simulink model "DDCU_wxt_v02_forA_LabviewV03"  (R2014a)
settings: Solver=FixedStepDiscrete  StartTime=0.0  StopTime=50  FixedStep=0.0005  RelTol=1e-3
InitFcn:
  | Veh_Par_wxt
values from neighbouring files (symbols this model uses):
  ag_thr = 0.4*g    (= 3.924)    [Veh_Par_wxt.m]
  B = 2.25    [Veh_Par_wxt.m]
  bra_pre_em = 12    [Veh_Par_wxt.m]
  bra_pre_gz2 = 12/3    (= 4)    [Veh_Par_wxt.m]
  bra_pre_gz34 = 12/3    (= 4)    [Veh_Par_wxt.m]
  bra_pre_yd = 12/2    (= 6)    [Veh_Par_wxt.m]
  brakepre_dem_data = [0 1 2 3 4 5 6 7 8 9 10 11 12]    [Veh_Par_wxt.m]
  brakeTrq_dem_data = [0 218.198 436.396 654.594 872.792 1090.99 1309.188 1527.386 1745.584 1963.782 2181.98 2400.178 2618.376]    [Veh_Par_wxt.m]
  bratrq_max = 4*2618.376    (= 10473.504)    [Veh_Par_wxt.m]
  eff_tran = 0.75    [Veh_Par_wxt.m]
  G = Mass*g    (= 36297)    [Veh_Par_wxt.m]
  kd1 = 1    [Veh_Par_wxt.m]
  kd2 = 1    [Veh_Par_wxt.m]
  kd3 = 1    [Veh_Par_wxt.m]
  ki1 = 1    [Veh_Par_wxt.m]
  ki2 = 1    [Veh_Par_wxt.m]
  ki3 = 1    [Veh_Par_wxt.m]
  kp1 = 1    [Veh_Par_wxt.m]
  kp2 = 1    [Veh_Par_wxt.m]
  kp3 = 1    [Veh_Par_wxt.m]
  L = 3.12    [Veh_Par_wxt.m]
  premax = 12    [Veh_Par_wxt.m]
  Radius = 0.20    (= 0.2)    [Veh_Par_wxt.m]
  s_opt_yi_add = 0.05    [Veh_Par_wxt.m]
  s_opt_zhuan_add = 0.05    [Veh_Par_wxt.m]
  spd_map_mot = [0 100 200 300 360 400 500 600 700 800 900]*tras_ratio    [Veh_Par_wxt.m]
  spdmax = 900*tras_ratio    (= 5580)    [Veh_Par_wxt.m]
  speed_thr_park = 5/3.6/Radius*30/pi    (= 66.3145596216)    [Veh_Par_wxt.m]
  tras_ratio = 6.2    [Veh_Par_wxt.m]
  trq_map_mot = [1200 1200 1200 1200 1200 1080 864 720 617 540 480]/tras_ratio    [Veh_Par_wxt.m]
  trqmax = 80    [Veh_Par_wxt.m]
  trqmax_yd = 200    [Veh_Par_wxt.m]
  v_thr1_b = 5    [Veh_Par_wxt.m]
  v_thr2_b = 20    [Veh_Par_wxt.m]
  v_thr_park = 5    [Veh_Par_wxt.m]
undefined symbols (not defined in the file or in its folder): DiscIntNeverNeededParam
libraries: simulink x231, ec5744lib x19
(part 11 of 16)

== system DDCU_wxt_v02_forA_LabviewV03/Data_Input/MCU2_VCU1/MCU2_VCU1/M3InputVolt_Sub ==
  In1 : Inport
  Out1 : Outport
  wires:
  In1/1 -> Out1/1

== system DDCU_wxt_v02_forA_LabviewV03/Data_Input/MCU2_VCU1/MCU2_VCU1/M3Speed_Sub ==
  In1 : Inport
  Out1 : Outport
  wires:
  In1/1 -> Out1/1

== system DDCU_wxt_v02_forA_LabviewV03/Data_Input/MCU2_VCU1/MCU2_VCU1/M3State_Sub ==
  In1 : Inport
  Out1 : Outport
  wires:
  In1/1 -> Out1/1

== system DDCU_wxt_v02_forA_LabviewV03/Data_Input/MCU2_VCU1/MCU2_VCU1/M3Torque_Sub ==
  In1 : Inport
  Out1 : Outport
  wires:
  In1/1 -> Out1/1

== system DDCU_wxt_v02_forA_LabviewV03/Data_Input/MCU2_VCU2/MCU2_VCU2/M3FaultCode_Sub ==
  In1 : Inport
  Out1 : Outport
  wires:
  In1/1 -> Out1/1

== system DDCU_wxt_v02_forA_LabviewV03/Data_Input/MCU2_VCU2/MCU2_VCU2/M3FaultGrade_Sub ==
  In1 : Inport
  Out1 : Outport
  wires:
  In1/1 -> Out1/1

== system DDCU_wxt_v02_forA_LabviewV03/Data_Input/MCU2_VCU2/MCU2_VCU2/M3IGBTTemp_Sub ==
  In1 : Inport
  Out1 : Outport
  wires:
  In1/1 -> Out1/1

== system DDCU_wxt_v02_forA_LabviewV03/Data_Input/MCU2_VCU2/MCU2_VCU2/M3Temp_Sub ==
  In1 : Inport
  Out1 : Outport
  wires:
  In1/1 -> Out1/1

== system DDCU_wxt_v02_forA_LabviewV03/Data_Input/MCU2_VCU2/MCU2_VCU2/M3TqLimit_Sub ==
  In1 : Inport
  Out1 : Outport
  wires:
  In1/1 -> Out1/1

== system DDCU_wxt_v02_forA_LabviewV03/Data_Input/MCU2_VCU3/MCU2_VCU3/M4Current_Sub ==
  In1 : Inport
  Out1 : Outport
  wires:
  In1/1 -> Out1/1

== system DDCU_wxt_v02_forA_LabviewV03/Data_Input/MCU2_VCU3/MCU2_VCU3/M4Direction_Sub ==
  In1 : Inport
  Out1 : Outport
  wires:
  In1/1 -> Out1/1

== system DDCU_wxt_v02_forA_LabviewV03/Data_Input/MCU2_VCU3/MCU2_VCU3/M4HeartBeat_Sub ==
  In1 : Inport
  Out1 : Outport
  wires:
  In1/1 -> Out1/1

== system DDCU_wxt_v02_forA_LabviewV03/Data_Input/MCU2_VCU3/MCU2_VCU3/M4InputVolt_Sub ==
  In1 : Inport
  Out1 : Outport
  wires:
  In1/1 -> Out1/1

== system DDCU_wxt_v02_forA_LabviewV03/Data_Input/MCU2_VCU3/MCU2_VCU3/M4Speed_Sub ==
  In1 : Inport
  Out1 : Outport
  wires:
  In1/1 -> Out1/1

== system DDCU_wxt_v02_forA_LabviewV03/Data_Input/MCU2_VCU3/MCU2_VCU3/M4State_Sub ==
  In1 : Inport
  Out1 : Outport
  wires:
  In1/1 -> Out1/1

== system DDCU_wxt_v02_forA_LabviewV03/Data_Input/MCU2_VCU3/MCU2_VCU3/M4Torque_Sub ==
  In1 : Inport
  Out1 : Outport
  wires:
  In1/1 -> Out1/1

== system DDCU_wxt_v02_forA_LabviewV03/Data_Input/MCU2_VCU4/MCU2_VCU4/M4FaultCode_Sub ==
  In1 : Inport
  Out1 : Outport
  wires:
  In1/1 -> Out1/1

== system DDCU_wxt_v02_forA_LabviewV03/Data_Input/MCU2_VCU4/MCU2_VCU4/M4FaultGrade_Sub ==
  In1 : Inport
  Out1 : Outport
  wires:
  In1/1 -> Out1/1

== system DDCU_wxt_v02_forA_LabviewV03/Data_Input/MCU2_VCU4/MCU2_VCU4/M4IGBTTemp_Sub ==
  In1 : Inport
  Out1 : Outport
  wires:
  In1/1 -> Out1/1

== system DDCU_wxt_v02_forA_LabviewV03/Data_Input/MCU2_VCU4/MCU2_VCU4/M4Temp_Sub ==
  In1 : Inport
  Out1 : Outport
  wires:
  In1/1 -> Out1/1

== system DDCU_wxt_v02_forA_LabviewV03/Data_Input/MCU2_VCU4/MCU2_VCU4/M4TqLimit_Sub ==
  In1 : Inport
  Out1 : Outport
  wires:
  In1/1 -> Out1/1

== system DDCU_wxt_v02_forA_LabviewV03/MainControl/mode_control/Park/park ==
  Signals : Inport
  1-D Lookup Table : Lookup_n-D  NumberOfTableDimensions=1  BreakpointsForDimension1=brakeTrq_dem_data  Table=brakepre_dem_data  InternalRulePriority=Speed  RndMeth=Simplest  InputSameDT=on
  1-D Lookup Table1 : Lookup_n-D  NumberOfTableDimensions=1  BreakpointsForDimension1=brakeTrq_dem_data  Table=brakepre_dem_data  InternalRulePriority=Speed  RndMeth=Simplest  InputSameDT=on
  Bus Selector : BusSelector  OutputSignals=YaoKong.brake_dem
  Constant : Constant  Value=bratrq_max
  Gain : Gain  Gain=1/2
  Gain1 : Gain  Gain=1/100
  Gain2 : Gain  Gain=1/2
  Gain3 : Gain  Gain=1/2
  HeartBeat : MATLAB Function  TreatAsAtomicUnit=on
  HeartBeat1 : MATLAB Function  TreatAsAtomicUnit=on
  Memory : Memory  InheritSampleTime=on
  Memory1 : Memory  InheritSampleTime=on
  Mux : Mux  Inputs=8
  Mux1 : Mux  Inputs=8
  Mux2 : Mux  Inputs=7
  Mux3 : Mux  Inputs=7
  Product : Product
  Saturation1 : Saturate  UpperLimit=premax  LowerLimit=0
  Saturation4 : Saturate  UpperLimit=premax  LowerLimit=0
  SpdLim_dem{,1..3} (4 alike) : Constant  Value=spdmax
  SpdSet_dem : Constant  Value=0
  SpdSet_dem1 : Constant
  SpdSet_dem2 : Constant
  SpdSet_dem3 : Constant
  TrqLim_dem{,1..3} (4 alike) : Constant
  TrqSet_dem{,1..3} (4 alike) : Constant  Value=0
  mot_drive : Constant
  mot_drive1 : Constant  Value=2
  mot_drive2 : Constant
  mot_drive3 : Constant  Value=2
  mot_enable{,1..3} (4 alike) : Constant  Value=2
  mot_mode{,1..3} (4 alike) : Constant
  mot_lf : Outport
  mot_lr : Outport  Port=2
  mot_rf : Outport  Port=3
  mot_rr : Outport  Port=4
  bra_pre_l : Outport  Port=5
  bra_pre_r : Outport  Port=6
  wires:
  mot_drive/1 -> Mux/3
  mot_mode/1 -> Mux/2
  TrqSet_dem/1 -> Mux/4
  mot_enable/1 -> Mux/1
  SpdSet_dem/1 -> Mux/5
  Mux/1 -> mot_lf/1
  Signals/1 -> Bus Selector/1
  1-D Lookup Table/1 -> Saturation4/1
  TrqLim_dem/1 -> Mux/6
  HeartBeat/1(life) -> Mux/8, Memory/1
  Memory/1 -> HeartBeat/1(life_pre)
  SpdLim_dem/1 -> Mux/7
  mot_drive1/1 -> Mux2/3
  mot_mode2/1 -> Mux2/2
  TrqSet_dem1/1 -> Mux2/4
  mot_enable2/1 -> Mux2/1
  SpdSet_dem1/1 -> Mux2/5
  Mux2/1 -> mot_rf/1
  TrqLim_dem1/1 -> Mux2/6
  SpdLim_dem1/1 -> Mux2/7
  mot_drive2/1 -> Mux1/3
  mot_mode1/1 -> Mux1/2
  TrqSet_dem2/1 -> Mux1/4
  mot_enable1/1 -> Mux1/1
  SpdSet_dem2/1 -> Mux1/5
  Mux1/1 -> mot_lr/1
  TrqLim_dem2/1 -> Mux1/6
  HeartBeat1/1(life) -> Mux1/8, Memory1/1
  Memory1/1 -> HeartBeat1/1(life_pre)
  SpdLim_dem2/1 -> Mux1/7
  mot_drive3/1 -> Mux3/3
  mot_mode3/1 -> Mux3/2
  TrqSet_dem3/1 -> Mux3/4
  mot_enable3/1 -> Mux3/1
  SpdSet_dem3/1 -> Mux3/5
  Mux3/1 -> mot_rr/1
  TrqLim_dem3/1 -> Mux3/6
  SpdLim_dem3/1 -> Mux3/7
  Constant/1 -> Product/1
  Bus Selector/1 -> Gain1/1  "<brake_dem>"
  Product/1 -> Gain/1
  Gain/1 -> Gain3/1, Gain2/1
  Gain1/1 -> Product/2
  Gain2/1 -> 1-D Lookup Table/1
  Gain3/1 -> 1-D Lookup Table1/1
  1-D Lookup Table1/1 -> Saturation1/1
  Saturation4/1 -> bra_pre_l/1
  Saturation1/1 -> bra_pre_r/1

== system DDCU_wxt_v02_forA_LabviewV03/MainControl/mode_control/backward/backward ==
  Signals : Inport
  Brake : Subsystem  TreatAsAtomicUnit=on
  Bus Selector : BusSelector  OutputSignals=YaoKong.acc_dem,YaoKong.brake_dem,YaoKong.HAC
  Constant : Constant  Value=0.15
  Drive : Subsystem  TreatAsAtomicUnit=on
  MATLAB Function : MATLAB Function  TreatAsAtomicUnit=on
  Multiport Switch : MultiPortSwitch  DataPortOrder=Zero-based contiguous  Inputs=2
  Switch Case1 : SwitchCase  CaseConditions={0,1}  ShowDefaultCase=off
  backward_dem : Outport
  wires:
  Constant/1 -> Brake/2(s_opt_yi)
  Brake/1(backward_dem) -> Multiport Switch/3
  Drive/1(backward_dem) -> Multiport Switch/2
  MATLAB Function/1(y) -> Switch Case1/1, Multiport Switch/1
  Switch Case1/2 -> Brake/Action
  Switch Case1/1 -> Drive/Action
  Multiport Switch/1 -> backward_dem/1
  Signals/1 -> Bus Selector/1, Drive/1(Signals), Brake/1(Signals)
  Bus Selector/1 -> MATLAB Function/1(acc_dem)  "<acc_dem>"
  Bus Selector/2 -> MATLAB Function/2(brake_dem)  "<brake_dem>"
  Bus Selector/3 -> MATLAB Function/3(HAC)  "<HAC>"

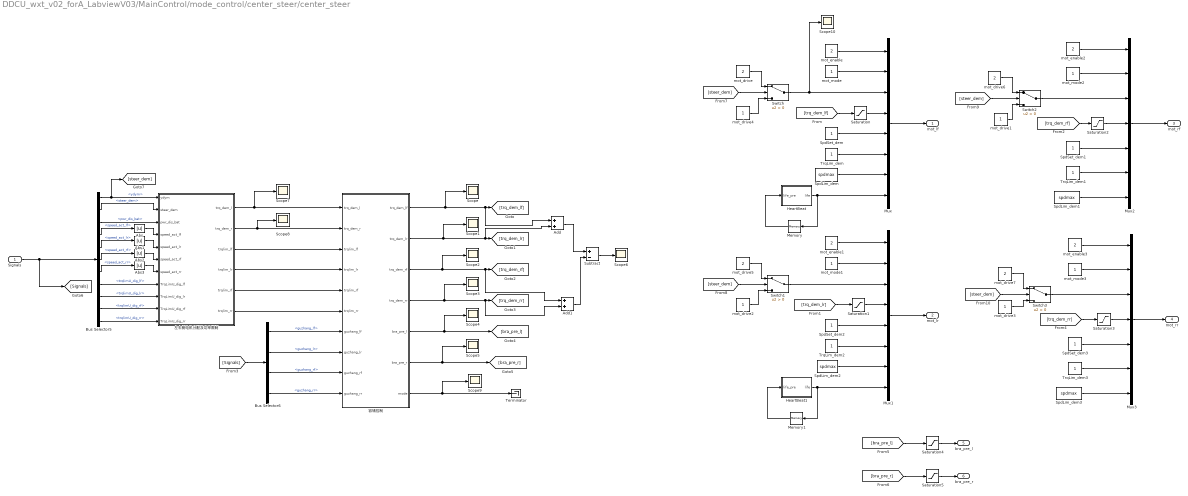
== system DDCU_wxt_v02_forA_LabviewV03/MainControl/mode_control/center_steer/center_steer ==
  Signals : Inport
  Abs{,1..3} (4 alike) : Abs
  Add : Sum
  Add1 : Sum
  Bus Selector5 : BusSelector  OutputSignals=ydym,YaoKong.steer_dem,Bat.pwr_dis_bat,DriveMotor.speed_act_lf,DriveMotor.speed_act_lr,DriveMotor.speed_act_rf,DriveMotor.speed_act_rr,DriveMotor.trqlimU_dig_lf,DriveMotor.trqlimU_dig_lr,DriveMotor.trqlimU_dig_rf,DriveMotor.trqlimU_dig_rr
  Bus Selector6 : BusSelector  OutputSignals=DriveMotor.guzhang_lf,DriveMotor.guzhang_lr,DriveMotor.guzhang_rf,DriveMotor.guzhang_rr
  HeartBeat : MATLAB Function  TreatAsAtomicUnit=on
  HeartBeat1 : MATLAB Function  TreatAsAtomicUnit=on
  Memory : Memory  InheritSampleTime=on
  Memory1 : Memory  InheritSampleTime=on
  Mux : Mux  Inputs=8
  Mux1 : Mux  Inputs=8
  Mux2 : Mux  Inputs=7
  Mux3 : Mux  Inputs=7
  Saturation{,1..3} (4 alike) : Saturate  UpperLimit=trqmax_yd  LowerLimit=0
  Saturation4 : Saturate  UpperLimit=premax  LowerLimit=0
  Saturation5 : Saturate  UpperLimit=premax  LowerLimit=0
  Scope{,1..10} (11 alike) : Scope
      Scope settings: SaveName=ScopeData47
      Scope1 settings: SaveName=ScopeData48
      Scope10 settings: SaveName=ScopeData58
      Scope2 settings: SaveName=ScopeData49
      Scope3 settings: SaveName=ScopeData50
      Scope4 settings: SaveName=ScopeData51
      Scope5 settings: SaveName=ScopeData52
      Scope6 settings: SaveName=ScopeData54
      Scope7 settings: SaveName=ScopeData55
      Scope8 settings: SaveName=ScopeData56
      Scope9 settings: SaveName=ScopeData57
  SpdLim_dem{,1..3} (4 alike) : Constant  Value=spdmax
  SpdSet_dem{,1..3} (4 alike) : Constant
  Subtract : Sum  Inputs=+-
  Switch{,1..3} (4 alike) : Switch  Criteria=u2 > Threshold
  Terminator : Terminator
  TrqLim_dem{,1..3} (4 alike) : Constant
  mot_drive{,5..7} (4 alike) : Constant  Value=2
  mot_drive{1..4} (4 alike) : Constant
  mot_enable{,1..3} (4 alike) : Constant  Value=2
  mot_mode{,1..3} (4 alike) : Constant
  容错控制 : Subsystem
  左右侧电机分配及功率限制 : Subsystem
  mot_lf : Outport
  mot_lr : Outport  Port=2
  mot_rf : Outport  Port=3
  mot_rr : Outport  Port=4
  bra_pre_l : Outport  Port=5
  bra_pre_r : Outport  Port=6
  wires:
  Signals/1 -> [Signals], Bus Selector5/1
  Bus Selector5/3 -> 左右侧电机分配及功率限制/3(pwr_dis_bat)  "<pwr_dis_bat>"
  Bus Selector5/4 -> Abs/1  "<speed_act_lf>"
  Bus Selector5/5 -> Abs1/1  "<speed_act_lr>"
  Bus Selector5/6 -> Abs2/1  "<speed_act_rf>"
  Bus Selector5/7 -> Abs3/1  "<speed_act_rr>"
  Bus Selector5/11 -> 左右侧电机分配及功率限制/11(TrqLimU_dig_rr)  "<trqlimU_dig_rr>"
  Bus Selector5/10 -> 左右侧电机分配及功率限制/10(TrqLimU_dig_rf)  "<trqlimU_dig_rf>"
  Bus Selector5/8 -> 左右侧电机分配及功率限制/8(TrqLimU_dig_lf)  "<trqlimU_dig_lf>"
  Bus Selector5/9 -> 左右侧电机分配及功率限制/9(TrqLimU_dig_lr)  "<trqlimU_dig_lr>"
  [Signals] -> Bus Selector6/1
  左右侧电机分配及功率限制/2(trq_dem_r) -> Scope8/1, 容错控制/2(trq_dem_r)
  左右侧电机分配及功率限制/1(trq_dem_l) -> Scope7/1, 容错控制/1(trq_dem_l)
  Bus Selector6/4 -> 容错控制/10(guzhang_rr)  "<guzhang_rr>"
  Bus Selector6/3 -> 容错控制/9(guzhang_rf)  "<guzhang_rf>"
  Bus Selector6/2 -> 容错控制/8(guzhang_lr)  "<guzhang_lr>"
  Bus Selector6/1 -> 容错控制/7(guzhang_lf)  "<guzhang_lf>"
  左右侧电机分配及功率限制/5(trqlim_rf) -> 容错控制/5(trqlim_rf)
  左右侧电机分配及功率限制/4(trqlim_lr) -> 容错控制/4(trqlim_lr)
  左右侧电机分配及功率限制/6(trqlim_rr) -> 容错控制/6(trqlim_rr)
  左右侧电机分配及功率限制/3(trqlim_lf) -> 容错控制/3(trqlim_lf)
  Bus Selector5/2 -> 左右侧电机分配及功率限制/2(steer_dem)  "<steer_dem>"
  容错控制/1(trq_dem_lf) -> Scope/1, Add/1, [trq_dem_lf]
  容错控制/3(trq_dem_rf) -> Scope2/1, Add1/1, [trq_dem_rf]
  容错控制/4(trq_dem_rr) -> Scope3/1, Add1/2, [trq_dem_rr]
  容错控制/5(bra_pre_l) -> Scope4/1, [bra_pre_l]
  容错控制/6(bra_pre_r) -> Scope5/1, [bra_pre_r]
  容错控制/2(trq_dem_lr) -> Scope1/1, Add/2, [trq_dem_lr]
  Switch/1 -> Scope10/1, Mux/3
  mot_mode/1 -> Mux/2
  [trq_dem_lf] -> Saturation/1
  mot_enable/1 -> Mux/1
  SpdSet_dem/1 -> Mux/5
  Mux/1 -> mot_lf/1
  TrqLim_dem/1 -> Mux/6
  HeartBeat/1(life) -> Mux/8, Memory/1
  Memory/1 -> HeartBeat/1(life_pre)
  SpdLim_dem/1 -> Mux/7
  Switch2/1 -> Mux2/3
  mot_mode2/1 -> Mux2/2
  [trq_dem_rf] -> Saturation2/1
  mot_enable2/1 -> Mux2/1
  SpdSet_dem1/1 -> Mux2/5
  Mux2/1 -> mot_rf/1
  TrqLim_dem1/1 -> Mux2/6
  SpdLim_dem1/1 -> Mux2/7
  Switch1/1 -> Mux1/3
  mot_mode1/1 -> Mux1/2
  [trq_dem_lr] -> Saturation1/1
  mot_enable1/1 -> Mux1/1
  SpdSet_dem2/1 -> Mux1/5
  Mux1/1 -> mot_lr/1
  TrqLim_dem2/1 -> Mux1/6
  HeartBeat1/1(life) -> Mux1/8, Memory1/1
  Memory1/1 -> HeartBeat1/1(life_pre)
  SpdLim_dem2/1 -> Mux1/7
  Switch3/1 -> Mux3/3
  mot_mode3/1 -> Mux3/2
  [trq_dem_rr] -> Saturation3/1
  mot_enable3/1 -> Mux3/1
  SpdSet_dem3/1 -> Mux3/5
  Mux3/1 -> mot_rr/1
  TrqLim_dem3/1 -> Mux3/6
  SpdLim_dem3/1 -> Mux3/7
  [bra_pre_l] -> Saturation4/1
  [bra_pre_r] -> Saturation5/1
  Saturation/1 -> Mux/4
  Saturation1/1 -> Mux1/4
  Saturation2/1 -> Mux2/4
  Saturation3/1 -> Mux3/4
  Saturation4/1 -> bra_pre_l/1
  Saturation5/1 -> bra_pre_r/1
  Add/1 -> Subtract/1
  Add1/1 -> Subtract/2
  Subtract/1 -> Scope6/1
  容错控制/7(mode) -> Terminator/1, Scope9/1
  Abs/1 -> 左右侧电机分配及功率限制/4(speed_act_lf)
  Abs1/1 -> 左右侧电机分配及功率限制/5(speed_act_lr)
  Abs2/1 -> 左右侧电机分配及功率限制/6(speed_act_rf)
  Abs3/1 -> 左右侧电机分配及功率限制/7(speed_act_rr)
  [steer_dem] -> Switch/2
  mot_drive4/1 -> Switch/3
  mot_drive/1 -> Switch/1
  [steer_dem] -> Switch1/2
  mot_drive5/1 -> Switch1/1
  mot_drive2/1 -> Switch1/3
  [steer_dem] -> Switch2/2
  mot_drive6/1 -> Switch2/1
  mot_drive1/1 -> Switch2/3
  [steer_dem] -> Switch3/2
  mot_drive7/1 -> Switch3/1
  mot_drive3/1 -> Switch3/3
  Bus Selector5/1 -> [steer_dem], 左右侧电机分配及功率限制/1(ydym)  "<ydym>"

== system DDCU_wxt_v02_forA_LabviewV03/MainControl/mode_control/emergency_stop/emergency_stop ==
  Signals : Inport
  Bus Selector : BusSelector  OutputSignals=YaoKong.brake_dem
  Constant : Constant  Value=bra_pre_em
  HeartBeat : MATLAB Function  TreatAsAtomicUnit=on
  HeartBeat1 : MATLAB Function  TreatAsAtomicUnit=on
  Memory : Memory  InheritSampleTime=on
  Memory1 : Memory  InheritSampleTime=on
  Mux : Mux  Inputs=8
  Mux1 : Mux  Inputs=8
  Mux2 : Mux  Inputs=7
  Mux3 : Mux  Inputs=7
  Saturation1 : Saturate  UpperLimit=premax  LowerLimit=0
  Saturation4 : Saturate  UpperLimit=premax  LowerLimit=0
  SpdLim_dem{,1..3} (4 alike) : Constant  Value=spdmax
  SpdSet_dem{,1..3} (4 alike) : Constant
  Terminator : Terminator
  TrqLim_dem{,1..3} (4 alike) : Constant
  TrqSet_dem{,1..3} (4 alike) : Constant  Value=0
  mot_drive : Constant
  mot_drive1 : Constant  Value=2
  mot_drive2 : Constant
  mot_drive3 : Constant  Value=2
  mot_enable{,1..3} (4 alike) : Constant  Value=2
  mot_mode{,1..3} (4 alike) : Constant
  mot_lf : Outport
  mot_lr : Outport  Port=2
  mot_rf : Outport  Port=3
  mot_rr : Outport  Port=4
  bra_pre_l : Outport  Port=5
  bra_pre_r : Outport  Port=6
  wires:
  mot_drive/1 -> Mux/3
  mot_mode/1 -> Mux/2
  TrqSet_dem/1 -> Mux/4
  mot_enable/1 -> Mux/1
  SpdSet_dem/1 -> Mux/5
  Mux/1 -> mot_lf/1
  Signals/1 -> Bus Selector/1
  Bus Selector/1 -> Terminator/1  "<brake_dem>"
  TrqLim_dem/1 -> Mux/6
  HeartBeat/1(life) -> Mux/8, Memory/1
  Memory/1 -> HeartBeat/1(life_pre)
  SpdLim_dem/1 -> Mux/7
  mot_drive1/1 -> Mux2/3
  mot_mode2/1 -> Mux2/2
  TrqSet_dem1/1 -> Mux2/4
  mot_enable2/1 -> Mux2/1
  SpdSet_dem1/1 -> Mux2/5
  Mux2/1 -> mot_rf/1
  TrqLim_dem1/1 -> Mux2/6
  SpdLim_dem1/1 -> Mux2/7
  mot_drive2/1 -> Mux1/3
  mot_mode1/1 -> Mux1/2
  TrqSet_dem2/1 -> Mux1/4
  mot_enable1/1 -> Mux1/1
  SpdSet_dem2/1 -> Mux1/5
  Mux1/1 -> mot_lr/1
  TrqLim_dem2/1 -> Mux1/6
  HeartBeat1/1(life) -> Mux1/8, Memory1/1
  Memory1/1 -> HeartBeat1/1(life_pre)
  SpdLim_dem2/1 -> Mux1/7
  mot_drive3/1 -> Mux3/3
  mot_mode3/1 -> Mux3/2
  TrqSet_dem3/1 -> Mux3/4
  mot_enable3/1 -> Mux3/1
  SpdSet_dem3/1 -> Mux3/5
  Mux3/1 -> mot_rr/1
  TrqLim_dem3/1 -> Mux3/6
  SpdLim_dem3/1 -> Mux3/7
  Constant/1 -> Saturation4/1, Saturation1/1
  Saturation4/1 -> bra_pre_l/1
  Saturation1/1 -> bra_pre_r/1

== system DDCU_wxt_v02_forA_LabviewV03/MainControl/mode_control/forward/forward ==
  note: 最佳滑移率
  note: 再加一些滤波的措施
  note: 坡道驻车，目前一直给1
  Signals : Inport
  Brake : Subsystem  TreatAsAtomicUnit=on
  Bus Selector : BusSelector  OutputSignals=YaoKong.acc_dem,YaoKong.brake_dem,YaoKong.HAC
  Constant : Constant  Value=0.15  SampleTime=-1
  Drive : Subsystem  TreatAsAtomicUnit=on
  MATLAB Function : MATLAB Function  TreatAsAtomicUnit=on
  Multiport Switch : MultiPortSwitch  DataPortOrder=Zero-based contiguous  Inputs=2
  Switch Case1 : SwitchCase  CaseConditions={0,1}  ShowDefaultCase=off
  forward_dem : Outport
  wires:
  Signals/1 -> Brake/1(Signals), Drive/1(Signals), Bus Selector/1
  Multiport Switch/1 -> forward_dem/1
  Switch Case1/1 -> Drive/Action
  Switch Case1/2 -> Brake/Action
  Bus Selector/1 -> MATLAB Function/1(acc_dem)  "<acc_dem>"
  MATLAB Function/1(y) -> Multiport Switch/1, Switch Case1/1
  Drive/1(forward_dem) -> Multiport Switch/2
  Brake/1(forward_dem) -> Multiport Switch/3
  Constant/1 -> Brake/2(s_opt_yi)
  Bus Selector/2 -> MATLAB Function/2(brake_dem)  "<brake_dem>"
  Bus Selector/3 -> MATLAB Function/3(HAC)  "<HAC>"

== system DDCU_wxt_v02_forA_LabviewV03/MainControl/mode_control/neutral/neutral ==
  Signals : Inport
  Bus Selector : BusSelector  OutputSignals=YaoKong.brake_dem
  Constant : Constant  Value=0
  Gain : Gain  Gain=1/2
  HeartBeat : MATLAB Function  TreatAsAtomicUnit=on
  HeartBeat1 : MATLAB Function  TreatAsAtomicUnit=on
  Memory : Memory  InheritSampleTime=on
  Memory1 : Memory  InheritSampleTime=on
  Mux : Mux  Inputs=8
  Mux1 : Mux  Inputs=8
  Mux2 : Mux  Inputs=7
  Mux3 : Mux  Inputs=7
  SpdLim_dem{,1..3} (4 alike) : Constant  Value=spdmax
  SpdSet_dem{,1..3} (4 alike) : Constant
  Terminator : Terminator
  TrqLim_dem{,1..3} (4 alike) : Constant
  TrqSet_dem{,1..3} (4 alike) : Constant  Value=0
  mot_drive : Constant
  mot_drive1 : Constant  Value=2
  mot_drive2 : Constant
  mot_drive3 : Constant  Value=2
  mot_enable{,1..3} (4 alike) : Constant  Value=2
  mot_mode{,1..3} (4 alike) : Constant
  mot_lf : Outport
  mot_lr : Outport  Port=2
  mot_rf : Outport  Port=3
  mot_rr : Outport  Port=4
  bra_pre_l : Outport  Port=5
  bra_pre_r : Outport  Port=6
  wires:
  mot_drive/1 -> Mux/3
  mot_mode/1 -> Mux/2
  TrqSet_dem/1 -> Mux/4
  mot_enable/1 -> Mux/1
  SpdSet_dem/1 -> Mux/5
  Mux/1 -> mot_lf/1
  Signals/1 -> Bus Selector/1
  Bus Selector/1 -> Gain/1  "<brake_dem>"
  TrqLim_dem/1 -> Mux/6
  HeartBeat/1(life) -> Mux/8, Memory/1
  Memory/1 -> HeartBeat/1(life_pre)
  SpdLim_dem/1 -> Mux/7
  mot_drive1/1 -> Mux2/3
  mot_mode2/1 -> Mux2/2
  TrqSet_dem1/1 -> Mux2/4
  mot_enable2/1 -> Mux2/1
  SpdSet_dem1/1 -> Mux2/5
  Mux2/1 -> mot_rf/1
  TrqLim_dem1/1 -> Mux2/6
  SpdLim_dem1/1 -> Mux2/7
  mot_drive2/1 -> Mux1/3
  mot_mode1/1 -> Mux1/2
  TrqSet_dem2/1 -> Mux1/4
  mot_enable1/1 -> Mux1/1
  SpdSet_dem2/1 -> Mux1/5
  Mux1/1 -> mot_lr/1
  TrqLim_dem2/1 -> Mux1/6
  HeartBeat1/1(life) -> Mux1/8, Memory1/1
  Memory1/1 -> HeartBeat1/1(life_pre)
  SpdLim_dem2/1 -> Mux1/7
  mot_drive3/1 -> Mux3/3
  mot_mode3/1 -> Mux3/2
  TrqSet_dem3/1 -> Mux3/4
  mot_enable3/1 -> Mux3/1
  SpdSet_dem3/1 -> Mux3/5
  Mux3/1 -> mot_rr/1
  TrqLim_dem3/1 -> Mux3/6
  SpdLim_dem3/1 -> Mux3/7
  Gain/1 -> Terminator/1
  Constant/1 -> bra_pre_r/1, bra_pre_l/1

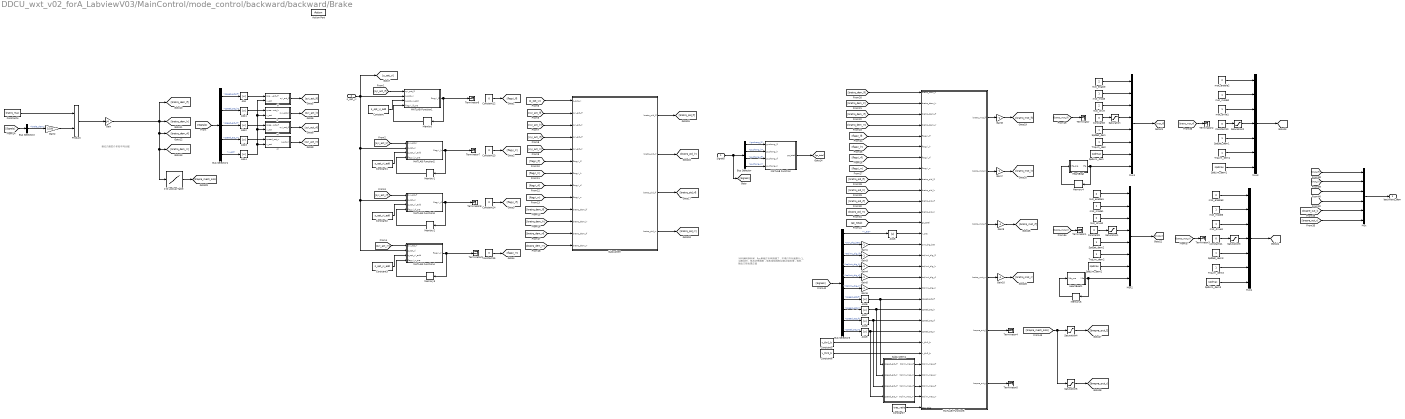
== system DDCU_wxt_v02_forA_LabviewV03/MainControl/mode_control/backward/backward/Brake ==
  note: 制动力矩四个车轮平均分配
  note: 当时编程序时候，fcn里面正负号搞错了，不得已在外面乘以-1，
      | 当制动时，电池功率限制，电机扭矩限制当做正值处理，电机
      | 输出力矩也是正值
  Signals : Inport
  s_opt_yi : Inport  Port=2
  Action Port : ActionPort  ActionType=case
  1-D Lookup Table : Lookup_n-D  NumberOfTableDimensions=1  BreakpointsForDimension1=brakeTrq_dem_data  Table=brakepre_dem_data  InternalRulePriority=Speed  RndMeth=Simplest  InputSameDT=on
  Abs{,1..9} (10 alike) : Abs
  Bus Selector : BusSelector  OutputSignals=DriveMotor.guzhang_lf,DriveMotor.guzhang_lr,DriveMotor.guzhang_rf,DriveMotor.guzhang_rr
  Bus Selector1 : BusSelector  OutputSignals=DriveMotor.speed_act_lf,DriveMotor.speed_act_lr,DriveMotor.speed_act_rf,DriveMotor.speed_act_rr,IMU.v_act
  Bus Selector2 : BusSelector  OutputSignals=YaoKong.brake_dem
  Bus Selector3 : BusSelector  OutputSignals=IMU.v_act,Bat.pwr_chg_bat,DriveMotor.trqlimL_dig_lf,DriveMotor.trqlimL_dig_lr,DriveMotor.trqlimL_dig_rf,DriveMotor.trqlimL_dig_rr,DriveMotor.speed_act_lf,DriveMotor.speed_act_lr,DriveMotor.speed_act_rf,DriveMotor.speed_act_rr
  Constant{,1..3} (4 alike) : Constant  Value=s_opt_yi_add
  Constant{8..15} (8 alike) : Constant  Value=0
  Constant4 : Constant  Value=bratrq_max
  Constant5 : Constant  Value=v_thr1_b
  Constant6 : Constant  Value=v_thr2_b
  Constant7 : Constant  Value=tras_ratio
  Gain : Gain  Gain=1/4
  Gain{1,3..10} (9 alike) : Gain  Gain=-1
  Gain2 : Gain  Gain=1/100
  HeartBeat : MATLAB Function  TreatAsAtomicUnit=on
  HeartBeat1 : MATLAB Function  TreatAsAtomicUnit=on
  MATLAB Function : MATLAB Function  TreatAsAtomicUnit=on
  MATLAB Function1 : MATLAB Function  TreatAsAtomicUnit=on
  MATLAB Function2 : MATLAB Function  TreatAsAtomicUnit=on
  MATLAB Function3 : MATLAB Function  TreatAsAtomicUnit=on
  MATLAB Function4 : MATLAB Function  TreatAsAtomicUnit=on
  MATLAB Function5 : MATLAB Function  TreatAsAtomicUnit=on
  Memory{,1..5} (6 alike) : Memory  InheritSampleTime=on
  Mux : Mux  Inputs=6
  Mux1 : Mux  Inputs=8
  Mux2 : Mux  Inputs=8
  Mux3 : Mux  Inputs=7
  Mux4 : Mux  Inputs=7
  Product : Product
  Saturation{,1..3} (4 alike) : Saturate  UpperLimit=0  LowerLimit=-trqmax
  Saturation4 : Saturate  UpperLimit=premax  LowerLimit=0
  Saturation5 : Saturate  UpperLimit=premax  LowerLimit=0
  SpdLim_dem{,1..3} (4 alike) : Constant  Value=spdmax
  SpdSet_dem{,1..3} (4 alike) : Constant
  Subsystem : Subsystem
  Subsystem1 : Subsystem
  Terminator{,1..9} (10 alike) : Terminator
  TrqLim_dem{,1..3} (4 alike) : Constant
  lf : Subsystem
  lr : Subsystem
  mot_drive : Constant  Value=2
  mot_drive1 : Constant
  mot_drive2 : Constant  Value=2
  mot_drive3 : Constant
  mot_enable{,1..3} (4 alike) : Constant  Value=2
  mot_mode{,1..3} (4 alike) : Constant
  rf : Subsystem
  rr : Subsystem
  backward_dem : Outport
  wires:
  Saturation5/1 -> [brapre_out_r]
  Saturation4/1 -> [brapre_out_l]
  Saturation3/1 -> Mux4/4
  Saturation2/1 -> Mux3/4
  Saturation1/1 -> Mux2/4
  Saturation/1 -> Mux1/4
  Gain10/1 -> [bratrq_mot_rr]
  Gain9/1 -> [bratrq_mot_rf]
  Gain7/1 -> [bratrq_mot_lr]
  Gain8/1 -> [bratrq_mot_lf]
  Constant5/1 -> MATLAB Function5/24(v_thr1_b)
  Subsystem1/1(trqlim_map_lf) -> MATLAB Function5/26(trqlim_map_lf)
  Subsystem1/2(trqlim_map_lr) -> MATLAB Function5/27(trqlim_map_lr)
  Subsystem1/3(trqlim_map_rf) -> MATLAB Function5/28(trqlim_map_rf)
  Subsystem1/4(trqlim_map_rr) -> MATLAB Function5/29(trqlim_map_rr)
  [gz_total] -> MATLAB Function5/13(gz_total)
  [bratrq_pid_rr] -> MATLAB Function5/12(bratrq_pid_rr)
  [bratrq_pid_rf] -> MATLAB Function5/11(bratrq_pid_rf)
  [bratrq_pid_lr] -> MATLAB Function5/10(bratrq_pid_lr)
  [bratrq_pid_lf] -> MATLAB Function5/9(bratrq_pid_lf)
  [flagyi_rr] -> MATLAB Function5/8(flagyi_rr)
  [flagyi_rf] -> MATLAB Function5/7(flagyi_rf)
  [flagyi_lr] -> MATLAB Function5/6(flagyi_lr)
  [flagyi_lf] -> MATLAB Function5/5(flagyi_lf)
  [bratrq_dem_rr] -> MATLAB Function5/4(bratrq_dem_rr)
  [bratrq_dem_lf] -> MATLAB Function5/1(bratrq_dem_lf)
  [bratrq_dem_rf] -> MATLAB Function5/3(bratrq_dem_rf)
  [bratrq_dem_lr] -> MATLAB Function5/2(bratrq_dem_lr)
  Gain6/1 -> MATLAB Function5/19(trqlimL_dig_rr)
  Gain5/1 -> MATLAB Function5/18(trqlimL_dig_rf)
  Gain4/1 -> MATLAB Function5/17(trqlimL_dig_lr)
  Gain3/1 -> MATLAB Function5/16(trqlimL_dig_lf)
  Gain1/1 -> MATLAB Function5/15(pwr_chg_bat)
  Constant6/1 -> MATLAB Function5/25(v_thr2_b)
  Product/1 -> Gain/1
  Bus Selector2/1 -> Gain2/1  "<brake_dem>"
  Gain2/1 -> Product/2
  Constant4/1 -> Product/1
  Bus Selector3/10 -> Abs9/1  "<speed_act_rr>"
  Bus Selector3/9 -> Abs8/1  "<speed_act_rf>"
  Bus Selector3/8 -> Abs7/1  "<speed_act_lr>"
  Bus Selector3/7 -> Abs6/1  "<speed_act_lf>"
  Bus Selector3/6 -> Gain6/1  "<trqlimL_dig_rr>"
  Bus Selector3/5 -> Gain5/1  "<trqlimL_dig_rf>"
  Bus Selector3/4 -> Gain4/1  "<trqlimL_dig_lr>"
  Bus Selector3/3 -> Gain3/1  "<trqlimL_dig_lf>"
  Bus Selector3/1 -> Abs5/1  "<v_act>"
  Bus Selector3/2 -> Gain1/1  "<pwr_chg_bat>"
  [Signals] -> Bus Selector3/1
  MATLAB Function5/6(brapre_out_r) -> Terminator5/1
  MATLAB Function5/5(brapre_out_l) -> Terminator4/1
  MATLAB Function5/4(bratrq_mot_rr) -> Gain10/1
  MATLAB Function5/2(bratrq_mot_lr) -> Gain7/1
  MATLAB Function5/3(bratrq_mot_rf) -> Gain9/1
  MATLAB Function5/1(bratrq_mot_lf) -> Gain8/1
  [brapre_out_r] -> Mux/6
  [brapre_out_l] -> Mux/5
  [mot_rr] -> Mux/4
  [mot_rf] -> Mux/3
  [mot_lr] -> Mux/2
  [mot_lf] -> Mux/1
  mot_drive/1 -> Mux1/3
  mot_mode/1 -> Mux1/2
  mot_enable/1 -> Mux1/1
  SpdSet_dem/1 -> Mux1/5
  Mux1/1 -> [mot_lf]
  TrqLim_dem/1 -> Mux1/6
  HeartBeat/1(life) -> Mux1/8, Memory4/1
  Memory4/1 -> HeartBeat/1(life_pre)
  SpdLim_dem/1 -> Mux1/7
  mot_drive1/1 -> Mux3/3
  mot_mode2/1 -> Mux3/2
  mot_enable2/1 -> Mux3/1
  SpdSet_dem1/1 -> Mux3/5
  Mux3/1 -> [mot_rf]
  TrqLim_dem1/1 -> Mux3/6
  SpdLim_dem1/1 -> Mux3/7
  mot_drive2/1 -> Mux2/3
  mot_mode1/1 -> Mux2/2
  Constant9/1 -> Saturation1/1
  mot_enable1/1 -> Mux2/1
  SpdSet_dem2/1 -> Mux2/5
  Mux2/1 -> [mot_lr]
  TrqLim_dem2/1 -> Mux2/6
  HeartBeat1/1(life) -> Mux2/8, Memory5/1
  Memory5/1 -> HeartBeat1/1(life_pre)
  SpdLim_dem2/1 -> Mux2/7
  mot_drive3/1 -> Mux4/3
  mot_mode3/1 -> Mux4/2
  Constant11/1 -> Saturation3/1
  mot_enable3/1 -> Mux4/1
  SpdSet_dem3/1 -> Mux4/5
  Mux4/1 -> [mot_rr]
  TrqLim_dem3/1 -> Mux4/6
  SpdLim_dem3/1 -> Mux4/7
  Mux/1 -> backward_dem/1
  Subsystem/4(bratrq_pid_rr) -> [bratrq_pid_rr]
  Subsystem/1(bratrq_pid_lf) -> [bratrq_pid_lf]
  Subsystem/3(bratrq_pid_rf) -> [bratrq_pid_rf]
  Subsystem/2(bratrq_pid_lr) -> [bratrq_pid_lr]
  [bratrq_dem_rr] -> Subsystem/13(bratrq_dem_rr)
  [bratrq_dem_rf] -> Subsystem/12(bratrq_dem_rf)
  [bratrq_dem_lr] -> Subsystem/11(bratrq_dem_lr)
  [bratrq_dem_lf] -> Subsystem/10(bratrq_dem_lf)
  Gain/1 -> [bratrq_dem_lf], [bratrq_dem_rf], 1-D Lookup Table/1, [bratrq_dem_rr], [bratrq_dem_lr]
  [Signals] -> Bus Selector2/1
  [flagyi_rr] -> Subsystem/9(flagyi_rr)
  [flagyi_lr] -> Subsystem/7(flagyi_lr)
  [flagyi_lf] -> Subsystem/6(flagyi_lf)
  [flagyi_rf] -> Subsystem/8(flagyi_rf)
  [syi_act_rr] -> Subsystem/5(syi_act_rr)
  [syi_act_rf] -> Subsystem/4(syi_act_rf)
  [syi_act_lr] -> Subsystem/3(syi_act_lr)
  [syi_act_lf] -> Subsystem/2(syi_act_lf)
  [s_opt_yi] -> Subsystem/1(s_opt_yi)
  [syi_act_rr] -> MATLAB Function4/1(syi_act_rr)
  [syi_act_rf] -> MATLAB Function3/1(syi_act_rf)
  [syi_act_lr] -> MATLAB Function2/1(syi_act_lr)
  [syi_act_lf] -> MATLAB Function1/1(syi_act_lf)
  rr/1(s_act_rr) -> [syi_act_rr]
  rf/1(syi_act_rf) -> [syi_act_rf]
  lf/1(syi_act_lf) -> [syi_act_lf]
  lr/1(syi_act_lr) -> [syi_act_lr]
  MATLAB Function1/1(flagyi_lf) -> Terminator6/1, Memory/1
  Memory/1 -> MATLAB Function1/4(flagyi_lf_pre)
  Constant/1 -> MATLAB Function1/3(s_opt_yi_add)
  MATLAB Function2/1(flagyi_lr) -> Terminator7/1, Memory1/1
  Memory1/1 -> MATLAB Function2/4(flagyi_lr_pre)
  Constant1/1 -> MATLAB Function2/3(s_opt_yi_add)
  MATLAB Function3/1(flagyi_rf) -> Terminator8/1, Memory2/1
  Memory2/1 -> MATLAB Function3/4(flagyi_rf_pre)
  Constant2/1 -> MATLAB Function3/3(s_opt_yi_add)
  s_opt_yi/1 -> [s_opt_yi], MATLAB Function1/2(s_opt_yi), MATLAB Function4/2(s_opt_yi), MATLAB Function3/2(s_opt_yi), MATLAB Function2/2(s_opt_yi)
  MATLAB Function4/1(flagyi_rr) -> Terminator9/1, Memory3/1
  Memory3/1 -> MATLAB Function4/4(flagyi_rr_pre)
  Constant3/1 -> MATLAB Function4/3(s_opt_yi_add)
  Bus Selector1/5 -> Abs4/1  "<v_act>"
  Bus Selector1/4 -> Abs3/1  "<speed_act_rr>"
  Bus Selector1/3 -> Abs2/1  "<speed_act_rf>"
  Bus Selector1/2 -> Abs1/1  "<speed_act_lr>"
  Bus Selector1/1 -> Abs/1  "<speed_act_lf>"
  [Signals] -> Bus Selector1/1
  MATLAB Function/1(gz_total) -> [gz_total]
  Bus Selector/1 -> MATLAB Function/1(guzhang_lf)  "<guzhang_lf>"
  Bus Selector/2 -> MATLAB Function/2(guzhang_lr)  "<guzhang_lr>"
  Bus Selector/4 -> MATLAB Function/4(guzhang_rr)  "<guzhang_rr>"
  Bus Selector/3 -> MATLAB Function/3(guzhang_rf)  "<guzhang_rf>"
  Signals/1 -> Bus Selector/1, [Signals]
  Abs/1 -> lf/1(speed_act_lf)
  Abs1/1 -> lr/1(speed_act_lr)
  Abs2/1 -> rf/1(speed_act_rf)
  Abs3/1 -> rr/1(speed_act_rr)
  Abs4/1 -> lf/2(v_act), lr/2(v_act), rf/2(v_act), rr/2(v_act)
  Abs5/1 -> MATLAB Function5/14(v_act)
  Abs6/1 -> MATLAB Function5/20(speed_act_lf), Subsystem1/1(speed_act_lf)
  Abs7/1 -> MATLAB Function5/21(speed_act_lr), Subsystem1/2(speed_act_lr)
  Abs8/1 -> MATLAB Function5/22(speed_act_rf), Subsystem1/3(speed_act_rf)
  Abs9/1 -> MATLAB Function5/23(speed_act_rr), Subsystem1/4(speed_act_rr)
  Constant7/1 -> MATLAB Function5/30(tras_ratio)
  1-D Lookup Table/1 -> [brapre_mech_solo]
  [brapre_mech_solo] -> Saturation5/1, Saturation4/1
  [bratrq_mot_lf] -> Terminator/1
  Constant8/1 -> Saturation/1
  [bratrq_mot_lr] -> Terminator1/1
  [bratrq_mot_rf] -> Terminator2/1
  Constant10/1 -> Saturation2/1
  [bratrq_mot_rr] -> Terminator3/1
  Constant12/1 -> [flagyi_lf]
  Constant13/1 -> [flagyi_lr]
  Constant14/1 -> [flagyi_rf]
  Constant15/1 -> [flagyi_rr]

== system DDCU_wxt_v02_forA_LabviewV03/MainControl/mode_control/backward/backward/Drive ==
  Signals : Inport
  Action Port : ActionPort  ActionType=case
  Abs{,1..18} (19 alike) : Abs
  Bus Selector : BusSelector  OutputSignals=YaoKong.acc_dem,IMU.v_act,DriveMotor.trqlimU_dig_lf,DriveMotor.trqlimU_dig_lr,DriveMotor.trqlimU_dig_rf,DriveMotor.trqlimU_dig_rr
  Bus Selector1 : BusSelector  OutputSignals=IMU.acc_y
  Bus Selector2 : BusSelector  OutputSignals=IMU.acc_y,YaoKong.steer_dem
  Bus Selector3 : BusSelector  OutputSignals=IMU.dis_east,IMU.dis_north,IMU.hangxiangangle
  Bus Selector4 : BusSelector  OutputSignals=IMU.v_act,DriveMotor.trqlimU_dig_lf,DriveMotor.trqlimU_dig_lr,DriveMotor.trqlimU_dig_rf,DriveMotor.trqlimU_dig_rr,YaoKong.steer_dem
  Bus Selector5 : BusSelector  OutputSignals=Bat.pwr_dis_bat,DriveMotor.speed_act_lf,DriveMotor.speed_act_lr,DriveMotor.speed_act_rf,DriveMotor.speed_act_rr,DriveMotor.trqlimU_dig_lf,DriveMotor.trqlimU_dig_lr,DriveMotor.trqlimU_dig_rf,DriveMotor.trqlimU_dig_rr
  Bus Selector6 : BusSelector  OutputSignals=DriveMotor.guzhang_lf,DriveMotor.guzhang_lr,DriveMotor.guzhang_rf,DriveMotor.guzhang_rr
  Bus Selector7 : BusSelector  OutputSignals=DriveMotor.speed_act_lf,DriveMotor.speed_act_lr,DriveMotor.speed_act_rf,DriveMotor.speed_act_rr,IMU.v_act,YaoKong.steer_dem,IMU.acc_y,YaoKong.brake_dem
  Bus Selector8 : BusSelector  OutputSignals=DriveMotor.speed_act_lf,DriveMotor.speed_act_lr,DriveMotor.speed_act_rf,DriveMotor.speed_act_rr
  Bus Selector9 : BusSelector  OutputSignals=DriveMotor.speed_act_lf,DriveMotor.speed_act_lr,DriveMotor.speed_act_rf,DriveMotor.speed_act_rr
  Constant : Constant  Value=ag_thr
  Constant1 : Constant
  MATLAB Function : MATLAB Function  TreatAsAtomicUnit=on
  Multiport Switch : MultiPortSwitch  DataPortOrder=Zero-based contiguous
  Scope : Scope
      settings: SaveName=ScopeData5
  Scope1 : Scope
      settings: SaveName=ScopeData6
  Scope2 : Scope
      settings: SaveName=ScopeData9
  Switch Case : SwitchCase  CaseConditions={0,1,2}  ShowDefaultCase=off
  Terminator : Terminator
  容错控制 : Subsystem
  左右侧电机分配及功率限制 : Subsystem
  目标直驶力矩确定模块 : Subsystem
  目标转向力矩确定模块 : Subsystem  TreatAsAtomicUnit=on
  直驶纠偏控制 : Subsystem  TreatAsAtomicUnit=on
  路面状况识别模块 : Subsystem
  车辆稳定性控制 : Subsystem  TreatAsAtomicUnit=on
  驱动防滑控制TCS : Subsystem
  backward_dem : Outport
  wires:
  路面状况识别模块/4(s_opt_yi) -> Terminator/1
  Constant1/1 -> 路面状况识别模块/1(In1)
  驱动防滑控制TCS/1(backward_dem) -> backward_dem/1
  [Signals] -> Bus Selector7/1
  Bus Selector7/8 -> 驱动防滑控制TCS/14(brake_dem)  "<brake_dem>"
  [s_opt_zhuan] -> 驱动防滑控制TCS/15(s_opt_zhuan)
  Bus Selector7/1 -> Abs6/1  "<speed_act_lf>"
  Bus Selector7/2 -> Abs7/1  "<speed_act_lr>"
  Bus Selector7/3 -> Abs8/1  "<speed_act_rf>"
  Bus Selector7/4 -> Abs9/1  "<speed_act_rr>"
  Bus Selector7/5 -> Abs10/1  "<v_act>"
  Bus Selector7/6 -> 驱动防滑控制TCS/12(steer_dem)  "<steer_dem>"
  Bus Selector7/7 -> 驱动防滑控制TCS/13(acc_y)  "<acc_y>"
  容错控制/4(trq_dem_rr) -> 驱动防滑控制TCS/4(trq_dem_rr)
  容错控制/3(trq_dem_rf) -> 驱动防滑控制TCS/3(trq_dem_rf)
  容错控制/2(trq_dem_lr) -> 驱动防滑控制TCS/2(trq_dem_lr)
  容错控制/6(bra_pre_r) -> 驱动防滑控制TCS/6(bra_pre_r)
  容错控制/5(bra_pre_l) -> 驱动防滑控制TCS/5(bra_pre_l)
  容错控制/1(trq_dem_lf) -> 驱动防滑控制TCS/1(trq_dem_lf)
  左右侧电机分配及功率限制/3(trqlim_lf) -> 容错控制/3(trqlim_lf)
  左右侧电机分配及功率限制/6(trqlim_rr) -> 容错控制/6(trqlim_rr)
  左右侧电机分配及功率限制/4(trqlim_lr) -> 容错控制/4(trqlim_lr)
  左右侧电机分配及功率限制/5(trqlim_rf) -> 容错控制/5(trqlim_rf)
  Bus Selector6/1 -> 容错控制/7(guzhang_lf)  "<guzhang_lf>"
  Bus Selector6/2 -> 容错控制/8(guzhang_lr)  "<guzhang_lr>"
  Bus Selector6/3 -> 容错控制/9(guzhang_rf)  "<guzhang_rf>"
  Bus Selector6/4 -> 容错控制/10(guzhang_rr)  "<guzhang_rr>"
  左右侧电机分配及功率限制/1(trq_dem_l) -> 容错控制/1(trq_dem_l)
  左右侧电机分配及功率限制/2(trq_dem_r) -> 容错控制/2(trq_dem_r)
  [Signals] -> Bus Selector6/1
  Bus Selector5/7 -> 左右侧电机分配及功率限制/9(TrqLimU_dig_lr)  "<trqlimU_dig_lr>"
  Bus Selector5/6 -> 左右侧电机分配及功率限制/8(TrqLimU_dig_lf)  "<trqlimU_dig_lf>"
  Bus Selector5/8 -> 左右侧电机分配及功率限制/10(TrqLimU_dig_rf)  "<trqlimU_dig_rf>"
  Bus Selector5/9 -> 左右侧电机分配及功率限制/11(TrqLimU_dig_rr)  "<trqlimU_dig_rr>"
  Bus Selector5/5 -> Abs5/1  "<speed_act_rr>"
  Bus Selector5/4 -> Abs4/1  "<speed_act_rf>"
  Bus Selector5/3 -> Abs3/1  "<speed_act_lr>"
  Bus Selector5/2 -> Abs2/1  "<speed_act_lf>"
  Bus Selector5/1 -> 左右侧电机分配及功率限制/3(pwr_dis_bat)  "<pwr_dis_bat>"
  [Signals] -> Bus Selector5/1
  Bus Selector2/1 -> MATLAB Function/1(acc_y)  "<acc_y>"
  Bus Selector4/3 -> 目标转向力矩确定模块/3(TrqLimU_dig_lr)  "<trqlimU_dig_lr>"
  Bus Selector4/2 -> 目标转向力矩确定模块/2(TrqLimU_dig_lf)  "<trqlimU_dig_lf>"
  Bus Selector4/1 -> Abs1/1  "<v_act>"
  Bus Selector4/6 -> 目标转向力矩确定模块/6(steer_dem)  "<steer_dem>"
  Bus Selector4/5 -> 目标转向力矩确定模块/5(TrqLimU_dig_rr)  "<trqlimU_dig_rr>"
  Bus Selector4/4 -> 目标转向力矩确定模块/4(TrqLimU_dig_rf)  "<trqlimU_dig_rf>"
  Bus Selector/6 -> 目标直驶力矩确定模块/6(TrqLimU_dig_rr)  "<trqlimU_dig_rr>"
  Bus Selector/5 -> 目标直驶力矩确定模块/5(TrqLimU_dig_rf)  "<trqlimU_dig_rf>"
  Bus Selector/3 -> 目标直驶力矩确定模块/3(TrqLimU_dig_lf)  "<trqlimU_dig_lf>"
  Bus Selector/4 -> 目标直驶力矩确定模块/4(TrqLimU_dig_lr)  "<trqlimU_dig_lr>"
  目标直驶力矩确定模块/1(Trq_line_dem) -> 左右侧电机分配及功率限制/1(Trq_line_dem)
  Multiport Switch/1 -> 左右侧电机分配及功率限制/2(delta_T_dem), Scope1/1
  Bus Selector3/3 -> 直驶纠偏控制/3(hangxiangangle)  "<hangxiangangle>"
  Bus Selector3/2 -> 直驶纠偏控制/2(dis_north)  "<dis_north>"
  Bus Selector3/1 -> 直驶纠偏控制/1(dis_east)  "<dis_east>"
  路面状况识别模块/3(s_opt_zhuan) -> [s_opt_zhuan]
  路面状况识别模块/2(f) -> [f]
  路面状况识别模块/1(umax) -> [umax]
  [f] -> 目标转向力矩确定模块/8(f)
  [umax] -> 目标转向力矩确定模块/7(umax)
  Constant/1 -> MATLAB Function/3(ag_thr)
  Bus Selector2/2 -> MATLAB Function/2(steer_dem)  "<steer_dem>"
  直驶纠偏控制/1(delta_Tjiupian) -> Multiport Switch/4
  目标转向力矩确定模块/1(delta_Tsteer_dem) -> Multiport Switch/3, Scope/1
  车辆稳定性控制/1(delta_Twending_dem) -> Multiport Switch/2
  Switch Case/3 -> 直驶纠偏控制/Action
  Switch Case/2 -> 目标转向力矩确定模块/Action
  Switch Case/1 -> 车辆稳定性控制/Action
  MATLAB Function/1(y) -> Switch Case/1, Multiport Switch/1, Scope2/1
  Bus Selector1/1 -> 车辆稳定性控制/1(acc_y)  "<acc_y>"
  Bus Selector/2 -> Abs/1  "<v_act>"
  Bus Selector/1 -> 目标直驶力矩确定模块/1(acc_dem)  "<acc_dem>"
  Signals/1 -> Bus Selector/1, Bus Selector2/1, Bus Selector1/1, Bus Selector3/1, Bus Selector4/1, [Signals]
  Abs/1 -> 目标直驶力矩确定模块/2(v_act)
  Abs1/1 -> 目标转向力矩确定模块/1(v_act)
  Abs2/1 -> 左右侧电机分配及功率限制/4(speed_act_lf)
  Abs3/1 -> 左右侧电机分配及功率限制/5(speed_act_lr)
  Abs4/1 -> 左右侧电机分配及功率限制/6(speed_act_rf)
  Abs5/1 -> 左右侧电机分配及功率限制/7(speed_act_rr)
  Abs6/1 -> 驱动防滑控制TCS/7(speed_act_lf)
  Abs7/1 -> 驱动防滑控制TCS/8(speed_act_lr)
  Abs8/1 -> 驱动防滑控制TCS/9(speed_act_rf)
  Abs9/1 -> 驱动防滑控制TCS/10(speed_act_rr)
  Abs10/1 -> 驱动防滑控制TCS/11(v_act)
  [Signals] -> Bus Selector8/1
  Bus Selector8/3 -> Abs13/1  "<speed_act_rf>"
  Bus Selector8/2 -> Abs12/1  "<speed_act_lr>"
  Bus Selector8/4 -> Abs14/1  "<speed_act_rr>"
  Bus Selector8/1 -> Abs11/1  "<speed_act_lf>"
  Abs11/1 -> 目标直驶力矩确定模块/7(speed_act_lf)
  Abs12/1 -> 目标直驶力矩确定模块/8(speed_act_lr)
  Abs13/1 -> 目标直驶力矩确定模块/9(speed_act_rf)
  Abs14/1 -> 目标直驶力矩确定模块/10(speed_act_rr)
  [Signals] -> Bus Selector9/1
  Bus Selector9/3 -> Abs17/1  "<speed_act_rf>"
  Bus Selector9/2 -> Abs16/1  "<speed_act_lr>"
  Bus Selector9/4 -> Abs18/1  "<speed_act_rr>"
  Abs15/1 -> 目标转向力矩确定模块/9(speed_act_lf)
  Abs16/1 -> 目标转向力矩确定模块/10(speed_act_lr)
  Abs17/1 -> 目标转向力矩确定模块/11(speed_act_rf)
  Abs18/1 -> 目标转向力矩确定模块/12(speed_act_rr)
  Bus Selector9/1 -> Abs15/1  "<speed_act_lf>"

== system DDCU_wxt_v02_forA_LabviewV03/MainControl/mode_control/center_steer/center_steer/容错控制 ==
  trq_dem_l : Inport
  trq_dem_r : Inport  Port=2
  trqlim_lf : Inport  Port=3
  trqlim_lr : Inport  Port=4
  trqlim_rf : Inport  Port=5
  trqlim_rr : Inport  Port=6
  guzhang_lf : Inport  Port=7
  guzhang_lr : Inport  Port=8
  guzhang_rf : Inport  Port=9
  guzhang_rr : Inport  Port=10
  Constant : Constant  Value=bra_pre_yd
  MATLAB Function : MATLAB Function  TreatAsAtomicUnit=on
  trq_dem_lf : Outport
  trq_dem_lr : Outport  Port=2
  trq_dem_rf : Outport  Port=3
  trq_dem_rr : Outport  Port=4
  bra_pre_l : Outport  Port=5
  bra_pre_r : Outport  Port=6
  mode : Outport  Port=7
  wires:
  guzhang_lr/1 -> MATLAB Function/8(guzhang_lr)
  guzhang_rf/1 -> MATLAB Function/9(guzhang_rf)
  guzhang_rr/1 -> MATLAB Function/10(guzhang_rr)
  guzhang_lf/1 -> MATLAB Function/7(guzhang_lf)
  trq_dem_r/1 -> MATLAB Function/2(trq_dem_r)
  trqlim_lr/1 -> MATLAB Function/4(trqlim_lr)
  trq_dem_l/1 -> MATLAB Function/1(trq_dem_l)
  trqlim_rf/1 -> MATLAB Function/5(trqlim_rf)
  trqlim_rr/1 -> MATLAB Function/6(trqlim_rr)
  trqlim_lf/1 -> MATLAB Function/3(trqlim_lf)
  MATLAB Function/1(trq_dem_lf) -> trq_dem_lf/1
  MATLAB Function/2(trq_dem_lr) -> trq_dem_lr/1
  MATLAB Function/3(trq_dem_rf) -> trq_dem_rf/1
  MATLAB Function/4(trq_dem_rr) -> trq_dem_rr/1
  MATLAB Function/5(bra_pre_l) -> bra_pre_l/1
  MATLAB Function/6(bra_pre_r) -> bra_pre_r/1
  Constant/1 -> MATLAB Function/11(bra_pre_yd)
  MATLAB Function/7(mode) -> mode/1

== system DDCU_wxt_v02_forA_LabviewV03/MainControl/mode_control/center_steer/center_steer/左右侧电机分配及功率限制 ==
  ydym : Inport
  steer_dem : Inport  Port=2
  pwr_dis_bat : Inport  Port=3
  speed_act_lf : Inport  Port=4
  speed_act_lr : Inport  Port=5
  speed_act_rf : Inport  Port=6
  speed_act_rr : Inport  Port=7
  TrqLimU_dig_lf : Inport  Port=8
  TrqLimU_dig_lr : Inport  Port=9
  TrqLimU_dig_rf : Inport  Port=10
  TrqLimU_dig_rr : Inport  Port=11
  Abs : Abs
  Add1 : Sum  Inputs=++++
  Add3 : Sum  Inputs=++++
  Constant : Constant  Value=9549
  Divide : Product  Inputs=**/
  Gain : Gain  Gain=1/4
  Gain1 : Gain  Gain=1/2
  Gain2 : Gain  Gain=1/100
  MinMax{,3..6} (5 alike) : MinMax  Inputs=2
  Product : Product
  mot_map{,1..3} (4 alike) : Lookup_n-D  NumberOfTableDimensions=1  BreakpointsForDimension1=spd_map_mot  Table=trq_map_mot  InternalRulePriority=Speed  RndMeth=Simplest  InputSameDT=on
  trq_dem_l : Outport
  trq_dem_r : Outport  Port=2
  trqlim_lf : Outport  Port=3
  trqlim_lr : Outport  Port=4
  trqlim_rf : Outport  Port=5
  trqlim_rr : Outport  Port=6
  wires:
  speed_act_rf/1 -> mot_map2/1, Add1/3
  speed_act_lr/1 -> mot_map1/1, Add1/2
  speed_act_rr/1 -> mot_map3/1, Add1/4
  speed_act_lf/1 -> mot_map/1, Add1/1
  Add1/1 -> Gain/1
  Constant/1 -> Divide/1
  pwr_dis_bat/1 -> Divide/2
  Gain/1 -> Divide/3
  mot_map3/1 -> MinMax3/1
  TrqLimU_dig_rr/1 -> MinMax3/2
  mot_map2/1 -> MinMax4/1
  TrqLimU_dig_rf/1 -> MinMax4/2
  mot_map1/1 -> MinMax5/1
  TrqLimU_dig_lr/1 -> MinMax5/2
  mot_map/1 -> MinMax6/1
  TrqLimU_dig_lf/1 -> MinMax6/2
  MinMax6/1 -> trqlim_lf/1, Add3/1
  MinMax5/1 -> trqlim_lr/1, Add3/2
  MinMax4/1 -> trqlim_rf/1, Add3/3
  MinMax3/1 -> trqlim_rr/1, Add3/4
  Divide/1 -> MinMax/1
  Add3/1 -> MinMax/2
  MinMax/1 -> Product/2
  Product/1 -> Gain1/1
  Gain1/1 -> trq_dem_r/1, trq_dem_l/1
  Gain2/1 -> Product/1
  Abs/1 -> Gain2/1
  ydym/1 -> Abs/1

== matlab function DDCU_wxt_v02_forA_LabviewV03/MainControl/mode_control/Park/park/HeartBeat ==
  data: life_pre input; life output
function life = fcn(life_pre)
%#codegen
life=life_pre+1;
if life>15
    life=0;
end
end

== matlab function DDCU_wxt_v02_forA_LabviewV03/MainControl/mode_switch/mode_switch ==
  data: mode_dem input; mode_dem_out output; brake_emerg input; speed_act_lf input; speed_act_lr input; speed_act_rf input; speed_act_rr input; v_act input; v_thr_park input; speed_thr_park input; mode_dem_out_pre input
function mode_dem_out = fcn(mode_dem,brake_emerg,speed_act_lf,speed_act_lr,speed_act_rf,speed_act_rr,v_act,v_thr_park,speed_thr_park,mode_dem_out_pre)
%#codegen
mode_dem_out=mode_dem_out_pre;

if mode_dem==0 && abs(v_act)<=v_thr_park && speed_act_lf<=speed_thr_park && speed_act_lr<=speed_thr_park && speed_act_rf<=speed_thr_park && speed_act_rr<=speed_thr_park && brake_emerg==0
    mode_dem_out=0; 
    %驻车
elseif mode_dem==1 && v_act>=-v_thr_park && speed_act_lf>=0 && speed_act_lr>=0 && speed_act_rf>=0 && speed_act_rr>=0 && brake_emerg==0
    mode_dem_out=1;
    %前进
elseif mode_dem==2 && brake_emerg==0
    mode_dem_out=2;
    %空挡
elseif mode_dem==3 && v_act<=v_thr_park && speed_act_lf>=0 && speed_act_lr>=0 && speed_act_rf>=0 && speed_act_rr>=0 && brake_emerg==0
    mode_dem_out=3;
    %后退
elseif mode_dem==4 && v_act<=v_thr_park &&  v_act>=-v_thr_park % && speed_act_lf==0 && speed_act_lr==0 && speed_act_rf==0 && speed_act_rr==0 && brake_emerg==0       
    mode_dem_out=4;
    %中心转向
elseif brake_emerg==1
    mode_dem_out=5;
% else
%     mode_dem_out=5;
end
end

== matlab function DDCU_wxt_v02_forA_LabviewV03/MainControl/mode_control/Park/park/HeartBeat1 ==
  data: life_pre input; life output
function life = fcn(life_pre)
%#codegen
life=life_pre+1;
if life>15
    life=0;
end
end

== matlab function DDCU_wxt_v02_forA_LabviewV03/MainControl/mode_control/forward/forward/Drive/目标转向力矩确定模块/MATLAB Function ==
  data: steer_dem input; Rturn_min output; G input; L input; umax input; B input; Tpeak_L input; Tpeak_R input; eff_tran input; Radius input; f input
function Rturn_min = fcn(steer_dem,G,L,umax,B,Tpeak_L,Tpeak_R,eff_tran,Radius,f)
%#codegen
if steer_dem>0
    Rturn_min=(G*L*umax/(4*B*(Tpeak_R*eff_tran/Radius-f*G/2))-0.925)/0.15*B;
else
    Rturn_min=(G*L*umax/(4*B*(Tpeak_L*eff_tran/Radius-f*G/2))-0.925)/0.15*B;
end
end

== matlab function DDCU_wxt_v02_forA_LabviewV03/MainControl/mode_control/forward/forward/Drive/目标转向力矩确定模块/MATLAB Function1 ==
  data: v_act input; Rturn_min_ag output; ag_thr input
function Rturn_min_ag = fcn(v_act,ag_thr)
%#codegen

    Rturn_min_ag=(v_act/3.6)^2/ag_thr;
end

== matlab function DDCU_wxt_v02_forA_LabviewV03/MainControl/mode_control/forward/forward/Drive/目标转向力矩确定模块/MATLAB Function2 ==
  data: umax input; delta_Tsteer_max output; G input; L input; B input; Radius input; Rturn_min_xy input
function delta_Tsteer_max = fcn(umax,G,L,B,Radius,Rturn_min_xy)
%#codegen

    delta_Fsteer_max=umax/(0.925+0.15*(Rturn_min_xy/B))*G*L/(2*B);
    delta_Tsteer_max=delta_Fsteer_max*Radius;
    
end

== matlab function DDCU_wxt_v02_forA_LabviewV03/MainControl/mode_control/forward/forward/Drive/MATLAB Function ==
  data: acc_y input; y output; steer_dem input; ag_thr input
function y = fcn(acc_y,steer_dem,ag_thr)
%#codegen
if abs(acc_y)>=ag_thr
    y=0;
    %侧向加速度超过阈值，需要进入稳定性控制区域
elseif steer_dem~=0
    y=1;
    %进入正常的转向力矩分配阶段
else 
    y=2;
end
end

== matlab function DDCU_wxt_v02_forA_LabviewV03/MainControl/mode_control/forward/forward/Drive/左右侧电机分配及功率限制/MATLAB Function ==
  data: trqlim_l input; trq_dem_l output; trq_dem_r output; trq_dem_l1 input; trqlim_r input; trq_dem_r1 input; delta_T_dem input
function [trq_dem_l,trq_dem_r] = fcn(trqlim_l,trq_dem_l1,trqlim_r,trq_dem_r1,delta_T_dem)
%#codegen
if trq_dem_l1==trqlim_l
    trq_dem_l=trq_dem_l1;
    trq_dem_r=trq_dem_l1+delta_T_dem;%这时候加的是负值
elseif trq_dem_r1==trqlim_r
    trq_dem_l=trq_dem_r1-delta_T_dem;
    trq_dem_r=trq_dem_r1;
    
else
    trq_dem_l=trq_dem_l1;
    trq_dem_r=trq_dem_r1;
end
% trq_dem_l=max(0,trq_dem_l);%限一下最小值，不要小于0
% trq_dem_r=max(0,trq_dem_r);
trq_dem_l=max(-trqlim_l,trq_dem_l);%小转向半径下，内侧履带是可能输出负转矩的，从地面吸收功率，给外侧，所以不能限到0，限到最大电机外特性负值
trq_dem_r=max(-trqlim_r,trq_dem_r);
end
